simulink model "SampleSERIAL"  (R2017a)
settings: Solver=VariableStepAuto  StartTime=0.0  StopTime=inf  RelTol=1e-3
libraries: martin_sean_RoombaLib x4, realtime_pacer_lib x1
settings Model: Creator=tuf53749  LastModifiedBy=Sean

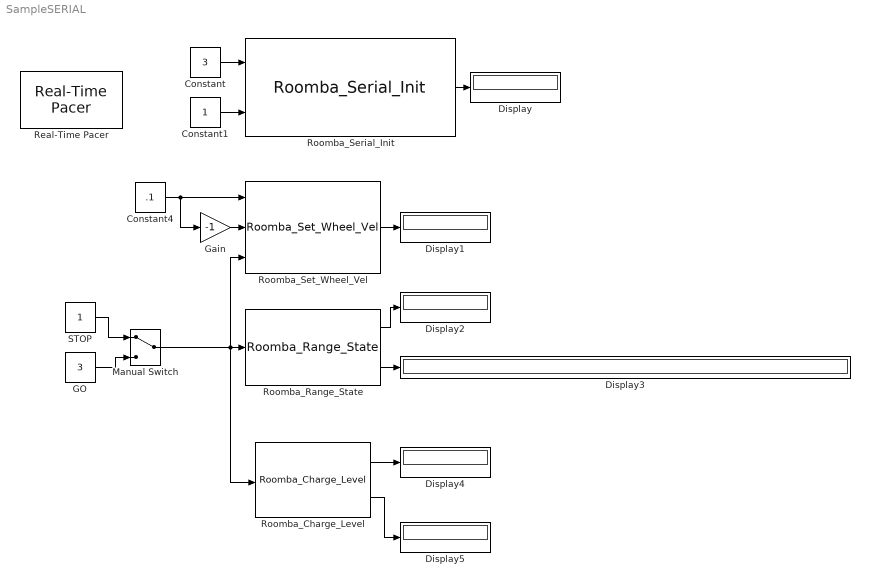
== system SampleSERIAL ==
  Constant : Constant  Value=3
  Constant1 : Constant
  Constant4 : Constant  Value=.1
  Display{,1..5} (6 alike) : Display
  GO : Constant  Value=3
  Gain : Gain  Gain=-1
  Manual Switch : ManualSwitch
  Real-Time Pacer : realtime_pacer_lib/Real-Time Pacer  simTimePerRealTime=1
  Roomba_Charge_Level : martin_sean_RoombaLib/Roomba_Charge_Level  Description=Returns the battery charge level on the Roomba as a percentage. Updates every 100 seconds.
  Roomba_Range_State : martin_sean_RoombaLib/Roomba_Range_State  Description=|
      | Returns [1x6] array containing the state of the six IR sensors on the front of the Roomba. A 
      | '1' indicates there is an object ahead and a '0' indicates no object.
  Roomba_Serial_Init : martin_sean_RoombaLib/Roomba_Serial_Init  Description=|  Priority=-1000
      | Initializes a serial connection to the Roomba. Takes the COM Port number and mode as inputs.
      | For instance, COM Port = 3 and Mode = 1 will set up a connection to the Roomba on COM3
      | and place it in 'full' mode.
      | 
      | A 0 is returned after successful initialization.
  Roomba_Set_Wheel_Vel : martin_sean_RoombaLib/Roomba_Set_Wheel_Vel  Description=|
      | Sets the right and left wheel velocities on the Roomba. The values are in meters/sec between 
      | [-0.5, 0.5]. Negative velocity is backwards.
  STOP : Constant
  wires:
  Constant/1 -> Roomba_Serial_Init/1
  Constant1/1 -> Roomba_Serial_Init/2
  Roomba_Serial_Init/1 -> Display/1
  STOP/1 -> Manual Switch/1
  GO/1 -> Manual Switch/2
  Constant4/1 -> Roomba_Set_Wheel_Vel/1, Gain/1
  Gain/1 -> Roomba_Set_Wheel_Vel/2
  Roomba_Set_Wheel_Vel/1 -> Display1/1
  Manual Switch/1 -> Roomba_Charge_Level/1, Roomba_Set_Wheel_Vel/3, Roomba_Range_State/1
  Roomba_Range_State/1 -> Display2/1
  Roomba_Range_State/2 -> Display3/1
  Roomba_Charge_Level/1 -> Display4/1
  Roomba_Charge_Level/2 -> Display5/1
